simulink model "mpc_demo_01"  (R2024b)
settings: Solver=ode4  StartTime=0.0  StopTime=20  FixedStep=0.01  RelTol=1e-3
settings Model: Creator=21192  LastModifiedBy=21192

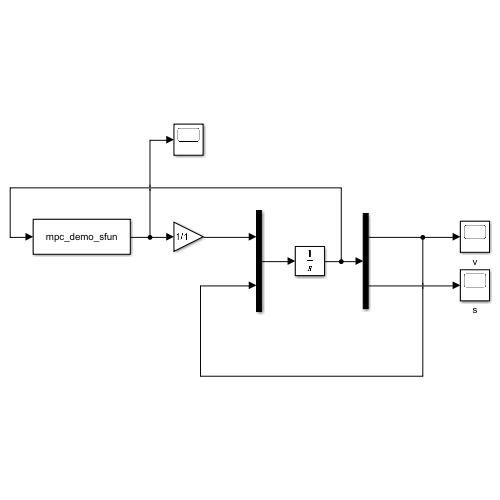
[thumbnail: Simulink's stored preview of the top-level diagram]
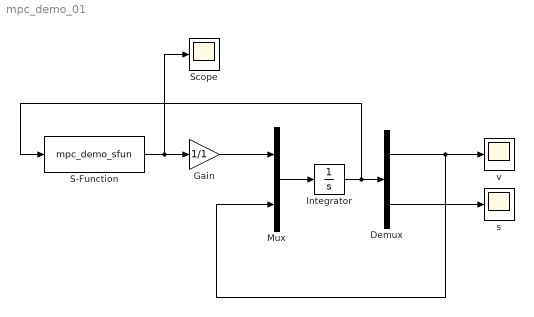
== system mpc_demo_01 ==
  Demux : Demux  Outputs=2
  Gain : Gain  Gain=1/1
  Integrator : Integrator  InitialCondition=[0;0]
  Mux : Mux  Inputs=2
  S-Function : S-Function  FunctionName=mpc_demo_sfun  SFunctionDeploymentMode=off  EnableBusSupport=off
  Scope : Scope
  s : Scope
  v : Scope
  wires:
  Integrator/1 -> S-Function/1, Demux/1
  S-Function/1 -> Scope/1, Gain/1
  Mux/1 -> Integrator/1
  Demux/1 -> v/1, Mux/2
  Gain/1 -> Mux/1
  Demux/2 -> s/1
